simulink subsystem "SimpleEngineSSC"  (R2024a)
settings: Solver=VariableStepAuto  StartTime=0.0  StopTime=10.0  RelTol=1e-3
undefined symbols (not defined in the file): Afr, BSFC, CrkAng, EngSpdOut, EngTrq, ExhManGasTemp, FuelFlw, FuelVolFlw, IntkPortFlw, NormAirChrg
libraries: fl_lib x3, nesl_utility x2, autolibsharedcommon x1, autolibpowerinfoutils x1, autolibsharedmappedengines x1, autolibutils x1
settings Model: ModifiedByFormat=The MathWorks, Inc.  Creator=The MathWorks, Inc.  LastModifiedBy=The MathWorks, Inc.
settings SolverCC: MaxZcPerStep=1
settings OptimizationCC: ReuseModelBlockBuffer=off
settings DebuggingCC: UnconnectedInputMsg=warning  UnconnectedOutputMsg=warning  UnconnectedLineMsg=warning
settings ModelReferenceCC: EnableRefExpFcnMdlSchedulingChecks=on
settings RTWCC: GPUComputeCapability=3.5  DLArmComputeVersion=19.05

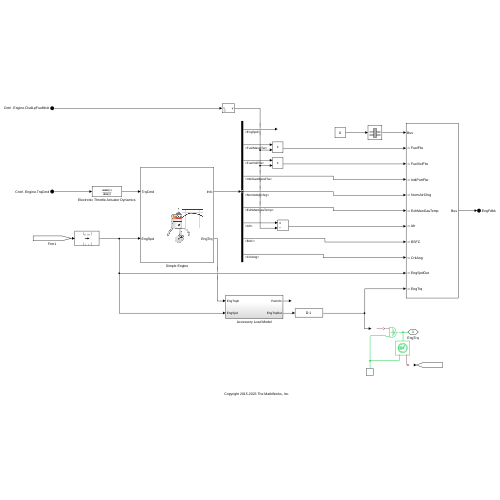
[thumbnail: Simulink's stored preview of the top-level diagram]
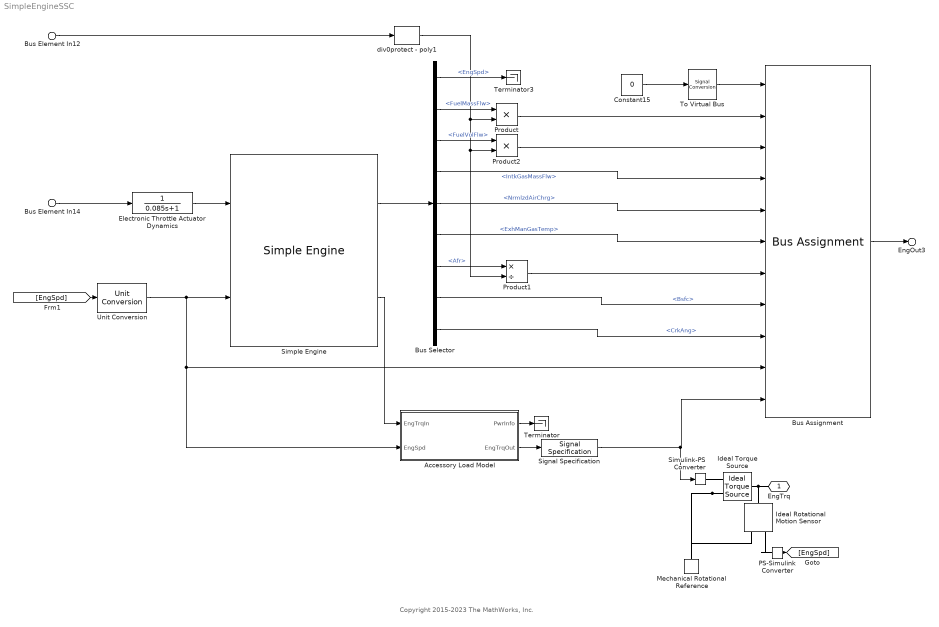
== system SimpleEngineSSC ==
  note: Copyright 2015-2023 The MathWorks, Inc.
  Bus Element In12 : Inport  PortName=Cntrl  Element=Engine.ClsdLpFuelMult
  Bus Element In14 : Inport  PortName=Cntrl  Element=Engine.TrqCmd
  Accessory Load Model : Subsystem
  Bus Assignment : BusAssignment  AssignedSignals=FuelFlw,FuelVolFlw,IntkPortFlw,NormAirChrg,ExhManGasTemp,Afr,BSFC,CrkAng,EngSpdOut,EngTrq
  Bus Selector : BusSelector  OutputSignals=EngSpd,FuelMassFlw,FuelVolFlw,IntkGasMassFlw,NrmlzdAirChrg,ExhManGasTemp,Afr,Bsfc,CrkAng
  Constant15 : Constant  Value=0  OutDataTypeStr=Bus: EngineBUS  SampleTime=Inf
  Electronic Throttle Actuator Dynamics : TransferFcn  Denominator=[0.085 1]
  Ideal Rotational Motion Sensor : fl_lib/Mechanical/Mechanical Sensors/Ideal Rotational Motion Sensor  reference=foundation.enum.MeasurementReference.difference  acceleration_port=false  velocity_port=true  position_port=false  wrap_angle=false  offset=0 rad
      settings: InternalSimscapePortConfiguration="{\"Bottom\":[],\"Left\":[{\"id\":\"R\",\"label\":\"R\",\"type\":\"foundation.mechanical.rotational.rotational\"}],\"Right\":[{\"id\":\"C\",\"label\":\"C\",\"type\":\"foundation.mechanical.rotational.rotational\"},{\"id\":\"W\",\"label\":\"W\",\"type\":\"output\"}],\"Top\":[]}"
  Ideal Torque Source : fl_lib/Mechanical/Mechanical Sources/Ideal Torque Source
  Mechanical Rotational Reference : fl_lib/Mechanical/Rotational Elements/Mechanical Rotational Reference
  PS-Simulink Converter : nesl_utility/PS-Simulink Converter  PhysicalDomain=network_engine_domain  SubClassName=ps_output  LeftPortType=input  RightPortType=output  PseudoPeriodic=off  Frequencies=[]  VectorFormat=inherit  Unit=rpm  AffineConversion=off
  Product : Product
  Product1 : Product  Inputs=*/
  Product2 : Product
  Signal Specification : SignalSpecification  Dimensions=1
  Simple Engine : autolibsharedmappedengines/Simple Engine  f_tqmax=PlntEngTqMax  f_tqmax_n_bpt=PlntEngTqMaxBpt  Lhv=PlntEngFuelLhv  Sg=PlntEngFuelSg  BsfcAvg=PlntEngBsfcAvg  aMode=6
  Simulink-PS Converter : nesl_utility/Simulink-PS Converter  PhysicalDomain=network_engine_domain  SubClassName=ps_input  LeftPortType=input  RightPortType=output  PseudoPeriodic=off  Frequencies=[]  NoiseDistribution=none  NoiseParameters=[]  Unit=N*m  AffineConversion=off  FilteringAndDerivatives=filter  SimscapeFilterOrder=1  InputFilterTimeConstant=0.001  UdotUserProvided=0
  Terminator : Terminator
  Terminator3 : Terminator
  To Virtual Bus : SignalConversion  ConversionOutput=Virtual bus  OverrideOpt=off
  Unit Conversion : UnitConversion
  div0protect - poly1 : autolibutils/div0protect - poly  thresh=0.01  ZeroCross1=off  aMode=6
  EngTrq : PMIOPort  Side=Right
  EngOut3 : Outport  PortName=EngFdbk
  wires:
  Simple Engine/2 -> Accessory Load Model/1(EngTrqIn)
  Bus Selector/9 -> Bus Assignment/9  "<CrkAng>"
  Bus Selector/1 -> Terminator3/1  "<EngSpd>"
  Product/1 -> Bus Assignment/2
  Bus Selector/6 -> Bus Assignment/6  "<ExhManGasTemp>"
  Bus Element In12/1 -> div0protect - poly1/1
  [EngSpd] -> Unit Conversion/1
  Accessory Load Model/2(EngTrqOut) -> Signal Specification/1
  Bus Selector/5 -> Bus Assignment/5  "<NrmlzdAirChrg>"
  div0protect - poly1/1 -> Product/2, Product1/2, Product2/2
  Accessory Load Model/1(PwrInfo) -> Terminator/1
  Bus Selector/3 -> Product2/1  "<FuelVolFlw>"
  Bus Element In14/1 -> Electronic Throttle Actuator Dynamics/1
  Product1/1 -> Bus Assignment/7
  Bus Selector/4 -> Bus Assignment/4  "<IntkGasMassFlw>"
  Bus Selector/7 -> Product1/1  "<Afr>"
  Bus Selector/2 -> Product/1  "<FuelMassFlw>"
  Electronic Throttle Actuator Dynamics/1 -> Simple Engine/1
  Product2/1 -> Bus Assignment/3
  Simple Engine/1 -> Bus Selector/1
  Bus Selector/8 -> Bus Assignment/8  "<Bsfc>"
  Unit Conversion/1 -> Accessory Load Model/2(EngSpd), Bus Assignment/10, Simple Engine/2
  To Virtual Bus/1 -> Bus Assignment/1
  Constant15/1 -> To Virtual Bus/1
  Bus Assignment/1 -> EngOut3/1
  PS-Simulink Converter/1 -> [EngSpd]
  Signal Specification/1 -> Simulink-PS Converter/1, Bus Assignment/11
  connections:
  Ideal Rotational Motion Sensor/LConn1 -- Ideal Torque Source/LConn1 -- EngTrq/RConn1
  Ideal Torque Source/RConn2 -- Ideal Rotational Motion Sensor/RConn1 -- Mechanical Rotational Reference/LConn1
  PS-Simulink Converter/LConn1 -- Ideal Rotational Motion Sensor/RConn2
  Simulink-PS Converter/RConn1 -- Ideal Torque Source/RConn1

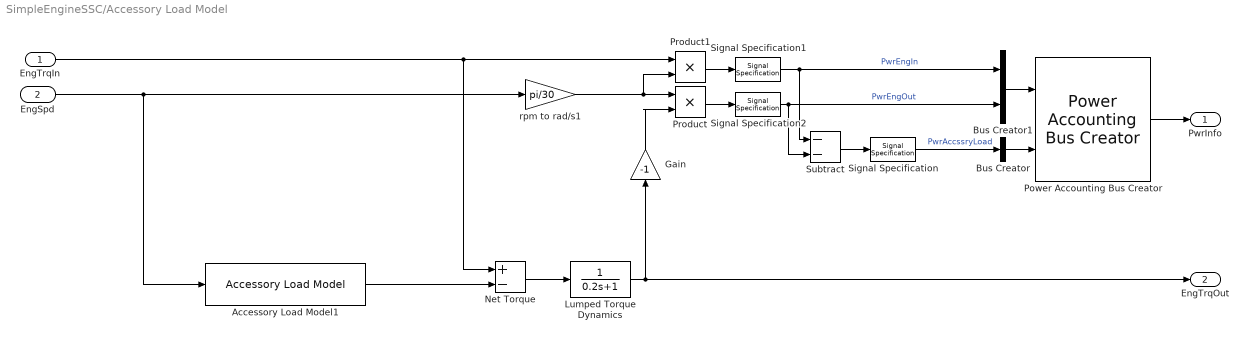
== system SimpleEngineSSC/Accessory Load Model ==
  EngTrqIn : Inport
  EngSpd : Inport  Port=2
  Accessory Load Model1 : autolibsharedcommon/Accessory Load Model  AccPwrTbl=PlntEngAccPwrTbl  AccSpdBpts=PlntEngAccSpdBpt  aMode=aMode
  Bus Creator : BusCreator  Inputs=1
  Bus Creator1 : BusCreator  Inputs=2
  Gain : Gain  Gain=-1
  Lumped Torque Dynamics : TransferFcn  Denominator=[0.2 1]
  Net Torque : Sum  Inputs=+-
  Power Accounting Bus Creator : autolibpowerinfoutils/Power Accounting Bus Creator  AssctBlkSelPopup=Parent  RefBlkName='libraryname/blkname'  PwrTrnsfrdCheckBox=on  PwrNotTrnsfrdCheckBox=on  PwrStoredCheckBox=off  aMode=6
  Product : Product
  Product1 : Product
  Signal Specification : SignalSpecification  Unit=W
  Signal Specification1 : SignalSpecification  Unit=W
  Signal Specification2 : SignalSpecification  Unit=W
  Subtract : Sum  Inputs=--
  rpm to rad/s1 : Gain  Gain=pi/30
  PwrInfo : Outport  VectorParamsAs1DForOutWhenUnconnected=off
  EngTrqOut : Outport  Port=2  Unit=N*m  VectorParamsAs1DForOutWhenUnconnected=off
  wires:
  Gain/1 -> Product/2
  Signal Specification2/1 -> Bus Creator1/2, Subtract/2  "PwrEngOut"
  Signal Specification1/1 -> Bus Creator1/1, Subtract/1  "PwrEngIn"
  rpm to rad/s1/1 -> Product/1, Product1/2
  Product1/1 -> Signal Specification1/1
  Product/1 -> Signal Specification2/1
  Power Accounting Bus Creator/1 -> PwrInfo/1
  Signal Specification/1 -> Bus Creator/1  "PwrAccssryLoad"
  Subtract/1 -> Signal Specification/1
  EngTrqIn/1 -> Net Torque/1, Product1/1
  Bus Creator1/1 -> Power Accounting Bus Creator/1
  Bus Creator/1 -> Power Accounting Bus Creator/2
  Net Torque/1 -> Lumped Torque Dynamics/1
  Lumped Torque Dynamics/1 -> Gain/1, EngTrqOut/1
  EngSpd/1 -> Accessory Load Model1/1, rpm to rad/s1/1
  Accessory Load Model1/1 -> Net Torque/2
